simulink model "youhua_1226"  (R2017b)
settings: Solver=ode1  StartTime=0.0  StopTime=Inf  FixedStep=0.0002  RelTol=1e-3
PreLoadFcn:
  | initFun_4P.m
PostLoadFcn:
  | , if any(exist('dsrtsu_mdlpostloadfcn', 'file') == [2, 3, 6]), try dsrtsu_mdlpostloadfcn('Execute', bdroot); catch fprintf('Error in PostLoadFcn (dsrtsu_mdlpostloadfcn) for model "%s":\n %s\n', bdroot, lasterr); end, end,
InitFcn:
  | initFun_4P
undefined symbols (not defined in the file): CMAES_B_initial, CMAES_C_initial, CMAES_chiN_initial, CMAES_counteval_initial, CMAES_D_initial, CMAES_eigeneval_initial, CMAES_invsqrtC_initial, CMAES_pc_initial, CMAES_ps_initial, CMAES_sigma_initial, CMAES_xmean_initial
libraries: rti1202lib_adc_class1 x20, simulink x8, dsparch4 x6, rti1202serlib x4, rti1202lib_dio_class1 x4, dsextras x3, rtiemclib x2, rti1202lib_dac_class1 x1, rtitasklib x1
(part 3 of 6)

== system youhua_1226/DSpace Sensor Raw Readings/Digital Pins ==
  Constant : Constant  OutDataTypeStr=boolean
  DIO_CLASS1_BIT_IN_BL2 : rti1202lib_dio_class1/DIO_CLASS1_BIT_IN_BL1  DSProperties=struct('RTI',struct('Version',uint32(1),'BlockType',struct('isSLSource',uint8(1),'isSLSink',uint8(0),'isHWSource',uint8(1),'isHWSink',uint8(0),'isSetup',uint8(0),'isInline',uint8(1),'isNonInline',uint8(0),'isInterrupt',uint8(0),'isChannelwise',uint8(1)),'IOBoardType',{{'DS120X','STD','DIOC1'}},'UnitType','BIT','Identifier','BITIN','DialogType','ML','BlockSet','NONE','SlaveProcessor','NONE'))  RTIBlockInterface=struct('OutputPortsWidth',int32(1),'OutputPortsDataType',{{'SS_BOOLEAN'}},'OutputPortsActive',1,'OutputPortsName',{{'Out'}},'BlockDisplay',{{['DIO CL1 BIT IN\nPort: 1\nChannel: 1\nNumber of channels: 1'],'center'}},'IconTransparency','on','InitLevel',3,'DialogFcn','rti120xstddioc1bitingui','BlockName',struct('Token',{{'DIO_CLASS1_BIT_IN_BL1'}}))  RTIBlockParameters=struct('PortNo',{{1,'OFF',[]}},'ChannelNo',{{1,'OFF',[]}},'ChannelNumOf',{{1,'OFF',[]}},'EnableNoiseFilter',{{0,'OFF',[0 1]}},'FilterInterval',{{'0','OFF',[0 0.01]}},'FilterIntervalCheck',{{logical(0),'OFF',[]}},'EnableEvent',{{0,'OFF',[0 1]}},'EventMode',{{1,'OFF',[1 3]}},'EventOnFalling',{{1,'OFF',[0 1]}},'EventOnRising',{{0,'OFF',[0 1]}},'EventDelay',{{'0','OFF',[0 1.34]}},'EventRate',{{'1','OFF',[1 256]}},'EventBuildCheck',{{logical(0),'OFF',[]}},'TriggerLine',{{1,'OFF',[1 16]}},'EventChannelNoIdx',{{1,'OFF',[1 16]}},'TLCFileName',{{'rti120xdio_c1_bit_in','OFF',[]}})  RTISFcnParameters=struct('PortNo','int16','ChannelNo','int16','ChannelNumOf','int16','EnableNoiseFilter','int16','FilterInterval','double','EnableEvent','int16','EventMode','int16','EventOnFalling','int16','EventOnRising','int16','EventDelay','double','EventRate','int16','TriggerLine','int16','EventChannelNoIdx','int16','TLCFileName','char')  RTIBlockParaDefault=struct('PortNo',1,'ChannelNo',1,'ChannelNumOf',1,'EnableNoiseFilter',0,'FilterInterval',0,'FilterIntervalCheck',0,'EnableEvent',0,'EventMode',1,'EventOnFalling',1,'EventOnRising',0,'EventDelay',0,'EventRate',1,'EventBuildCheck',0,'TriggerLine',1,'EventChannelNoIdx',1,'TLCFileName','rti120xdio_c1_bit_in')
  DIO_CLASS1_BIT_OUT_BL1 : rti1202lib_dio_class1/DIO_CLASS1_BIT_OUT_BL1  DSProperties=struct('RTI',struct('Version',uint32(1),'BlockType',struct('isSLSource',uint8(0),'isSLSink',uint8(1),'isHWSource',uint8(0),'isHWSink',uint8(1),'isSetup',uint8(0),'isInline',uint8(1),'isNonInline',uint8(0),'isInterrupt',uint8(0),'isChannelwise',uint8(1)),'IOBoardType',{{'DS120X','STD','DIOC1'}},'UnitType','BIT','Identifier','BITOUT','DialogType','ML','BlockSet','NONE','SlaveProcessor','NONE'))  RTIBlockInterface=struct('InputPortsWidth',int32(1),'InputPortsActive',1,'InputPortsDataType',{{'SS_BOOLEAN'}},'InputPortsName',{{'In'}},'BlockDisplay',{{['DIO CL1 BIT OUT\nPort: 1\nChannel: 2\nNumber of channels: 1'],'center\'}},'IconTransparency','on','InitLevel',3,'DialogFcn','rti120xstddioc1bitoutgui','BlockName',struct('Token',{{'DIO_CLASS1_BIT_OUT_BL1'}}))  RTIBlockParameters=struct('PortNo',{{1,'OFF',[]}},'ChannelNo',{{2,'OFF',[]}},'ChannelNumOf',{{1,'OFF',[]}},'HighLevel',{{3,'OFF',[1 3]}},'OutputStateInit',{{zeros(1,16),'OFF',[0 1]}},'OutputStateTerm',{{zeros(1,16),'OFF',[0 1]}},'TerminationMode',{{0,'OFF',[0 1]}},'OutputStateTermValidate',{{0,'OFF',[0 1]}},'OutputStateInitSetAll',{{0,'OFF',[0 1]}},'OutputStateTermSetAll',{{0,'OFF',[0 1]}},'EnableEvent',{{0,'OFF',[0 1]}},'EventMode',{{1,'OFF',[1 3]}},'EventOnFalling',{{1,'OFF',[0 1]}},'EventOnRising',{{0,'OFF',[0 1]}},'EventDelay',{{'0','OFF',[0 1.34]}},'EventRate',{{'1','OFF',[1 256]}},'EventBuildCheck',{{logical(0),'OFF',[]}},'TriggerLine',{{1,'OFF',[1 16]}},'EventChannelNoIdx',{{1,'OFF',[1 16]}},'TLCFileName',{{'rti120xdio_c1_bit_out','OFF',[]}})  RTISFcnParameters=struct('PortNo','int16','ChannelNo','int16','ChannelNumOf','int16','HighLevel','int16','OutputStateInit','int16','OutputStateTerm','int16','TerminationMode','int16','OutputStateTermValidate','int16','EnableEvent','int16','EventMode','int16','EventOnFalling','int16','EventOnRising','int16','EventDelay','double','EventRate','int16','TriggerLine','int16','EventChannelNoIdx','int16','TLCFileName','char')  RTIBlockParaDefault=struct('PortNo',1,'ChannelNo',1,'ChannelNumOf',1,'HighLevel',1,'OutputStateInit',zeros(1,16),'OutputStateTerm',zeros(1,16),'TerminationMode',0,'OutputStateTermValidate',0,'OutputStateInitSetAll',0,'OutputStateTermSetAll',0,'EnableEvent',0,'EventMode',1,'EventOnFalling',1,'EventOnRising',0,'EventDelay',0,'EventRate',1,'EventBuildCheck',0,'TriggerLine',1,'EventChannelNoIdx',1,'TLCFileName','rti120xdio_c1_bit_out')
  Data Type Conversion : DataTypeConversion  OutDataTypeStr=double
  Out1 : Outport
  wires:
  DIO_CLASS1_BIT_IN_BL2/1 -> Data Type Conversion/1
  Constant/1 -> DIO_CLASS1_BIT_OUT_BL1/1
  Data Type Conversion/1 -> Out1/1

== system youhua_1226/DSpace Sensor Raw Readings/Encoder Readings ==
  EMC_ENCODER_BL2 : rtiemclib/EMC_ENCODER_BL1  DSProperties=struct('RTI',struct('Version',uint32(2),'BlockType',struct('isSLSource',uint8(1),'isSLSink',uint8(0),'isHWSource',uint8(1),'isHWSink',uint8(0),'isSetup',uint8(0),'isInline',uint8(1),'isNonInline',uint8(0),'isInterrupt',uint8(0),'isChannelwise',uint8(1)),'IOBoardType','DSEMC','UnitType','ENCODER','Identifier','ENCODER','DialogType','ML','BlockSet','RTIEMC','SlaveProcessor','NONE'))  RTIBlockInterface=struct('OutputPortsWidth',int32([1 1 1]),'OutputPortsActive',int32([1 1 0]),'OutputPortsName',{{'Position','Speed',['Index Detected']}},'OutputPortsDataType',{{'SS_DOUBLE','SS_DOUBLE','SS_BOOLEAN'}},'InitLevel',3,'IconTransparency','on','BlockDisplay',{{['EMC Encoder\nUnit: 1\nDIO class: 2\nPort: 1\nChannel: 1'],'center'}},'DialogFcn','rtiemcencodergui','BlockName',struct('Token',{{'EMC_ENCODER_BL1'}}))  RTIBlockParameters=struct('UnitNo',{{1,'OFF',[1 6]}},'DioClassNo',{{2,'OFF',[1 2]}},'PortNo',{{1,'OFF',[1 1]}},'ChannelNo',{{1,'OFF',[1 11]}},'HwSignalPin',{{['DIO1 ch1'],'OFF',[]}},'HwRefPin',{{'GND','OFF',[]}},'EnablePosMeasurement',{{1,'OFF',[0 1]}},'IndexSetMode',{{1,'OFF',[1 3]}},'EnableMinSpeed',{{1,'OFF',[0 1]}},'NumOfLines',{{'1250','OFF',[1 2097152]}},'InitAngleValue',{{'60','OFF',[0 359.99999]}},'IndexAngleValue',{{'0','OFF',[0 359.99999]}},'MinSpeedAngleValue',{{'45','OFF',[0.04 10000]}},'MinPosValue',{{'-125000','OFF',[-2097152 2097150.75]}},'MaxPosValue',{{'125000','OFF',[-2097151 2097151.75]}},'InitPosValue',{{'0','OFF',[-2097152 2097151.75]}},'IndexPosValue',{{'0','OFF',[-2097152 2097151.75]}},'MinSpeedPosValue',{{'1','OFF',[1 1000000]}},'IndexGateMode',{{1,'OFF',[0 1]}},'EnableNoiseFilter',{{0,'OFF',[0 1]}},'FilterInterval',{{'0','OFF',[0 0.01]}},'IndexDetectedOutPortMode',{{1,'OFF',[0 1]}},'BuildCheckAngleMeasurement',{{0,'OFF',[0 1]}},'BuildCheckAngleIndexMode',{{0,'OFF',[0 1]}},'BuildCheckPosIndexMode',{{0,'OFF',[0 1]}},'BuildCheckAngleMinSpeed',{{0,'OFF',[0 1]}},'BuildCheckPosMinSpeed',{{1,'OFF',[0 1]}},'TLCFileName',{{'rtiemcencoder','OFF',[]}})  RTISFcnParameters=struct('UnitNo','int32','DioClassNo','int32','PortNo','int32','ChannelNo','int32','EnablePosMeasurement','int32','IndexSetMode','int32','IndexDetectedOutPortMode','int32','EnableMinSpeed','int32','NumOfLines','uint32','InitAngleValue','double','IndexAngleValue','double','MinSpeedAngleValue','double','MinPosValue','double','MaxPosValue','double','InitPosValue','double','IndexPosValue','double','MinSpeedPosValue','double','IndexGateMode','int32','EnableNoiseFilter','int32','FilterInterval','double','TLCFileName','char')  RTIBlockParaDefault=struct('UnitNo',1,'DioClassNo',1,'PortNo',1,'ChannelNo',1,'HwSignalPin',['DIO1 ch1'],'HwRefPin','GND','EnablePosMeasurement',0,'IndexSetMode',1,'EnableMinSpeed',0,'NumOfLines',1024,'InitAngleValue',60,'IndexAngleValue',0,'MinSpeedAngleValue',45,'MinPosValue',0,'MaxPosValue',1023.75,'InitPosValue',0,'IndexPosValue',0,'MinSpeedPosValue',100,'IndexGateMode',0,'EnableNoiseFilter',0,'FilterInterval',0,'IndexDetectedOutPortMode',0,'BuildCheckAngleMeasurement',1,'BuildCheckAngleIndexMode',0,'BuildCheckPosIndexMode',0,'BuildCheckAngleMinSpeed',0,'BuildCheckPosMinSpeed',0,'TLCFileName','rtiemcencoder')
      settings: SourceProductName=dSPACE RTI Electric Motor Control Blockset
  EMC_ENCODER_BL4 : rtiemclib/EMC_ENCODER_BL1  DSProperties=struct('RTI',struct('Version',uint32(2),'BlockType',struct('isSLSource',uint8(1),'isSLSink',uint8(0),'isHWSource',uint8(1),'isHWSink',uint8(0),'isSetup',uint8(0),'isInline',uint8(1),'isNonInline',uint8(0),'isInterrupt',uint8(0),'isChannelwise',uint8(1)),'IOBoardType','DSEMC','UnitType','ENCODER','Identifier','ENCODER','DialogType','ML','BlockSet','RTIEMC','SlaveProcessor','NONE'))  RTIBlockInterface=struct('OutputPortsWidth',int32([1 1 1]),'OutputPortsActive',int32([1 1 0]),'OutputPortsName',{{'Position','Speed',['Index Detected']}},'OutputPortsDataType',{{'SS_DOUBLE','SS_DOUBLE','SS_BOOLEAN'}},'InitLevel',3,'IconTransparency','on','BlockDisplay',{{['EMC Encoder\nUnit: 3\nDIO class: 2\nPort: 1\nChannel: 5'],'center'}},'DialogFcn','rtiemcencodergui','BlockName',struct('Token',{{'EMC_ENCODER_BL1'}}))  RTIBlockParameters=struct('UnitNo',{{3,'OFF',[1 6]}},'DioClassNo',{{2,'OFF',[1 2]}},'PortNo',{{1,'OFF',[1 1]}},'ChannelNo',{{5,'OFF',[1 11]}},'HwSignalPin',{{['DIO1 ch1'],'OFF',[]}},'HwRefPin',{{'GND','OFF',[]}},'EnablePosMeasurement',{{1,'OFF',[0 1]}},'IndexSetMode',{{1,'OFF',[1 3]}},'EnableMinSpeed',{{1,'OFF',[0 1]}},'NumOfLines',{{'1250','OFF',[1 2097152]}},'InitAngleValue',{{'60','OFF',[0 359.99999]}},'IndexAngleValue',{{'0','OFF',[0 359.99999]}},'MinSpeedAngleValue',{{'45','OFF',[0.04 10000]}},'MinPosValue',{{'-125000','OFF',[-2097152 2097150.75]}},'MaxPosValue',{{'125000','OFF',[-2097151 2097151.75]}},'InitPosValue',{{'0','OFF',[-2097152 2097151.75]}},'IndexPosValue',{{'0','OFF',[-2097152 2097151.75]}},'MinSpeedPosValue',{{'1','OFF',[1 1000000]}},'IndexGateMode',{{1,'OFF',[0 1]}},'EnableNoiseFilter',{{0,'OFF',[0 1]}},'FilterInterval',{{'0','OFF',[0 0.01]}},'IndexDetectedOutPortMode',{{1,'OFF',[0 1]}},'BuildCheckAngleMeasurement',{{0,'OFF',[0 1]}},'BuildCheckAngleIndexMode',{{0,'OFF',[0 1]}},'BuildCheckPosIndexMode',{{0,'OFF',[0 1]}},'BuildCheckAngleMinSpeed',{{0,'OFF',[0 1]}},'BuildCheckPosMinSpeed',{{1,'OFF',[0 1]}},'TLCFileName',{{'rtiemcencoder','OFF',[]}})  RTISFcnParameters=struct('UnitNo','int32','DioClassNo','int32','PortNo','int32','ChannelNo','int32','EnablePosMeasurement','int32','IndexSetMode','int32','IndexDetectedOutPortMode','int32','EnableMinSpeed','int32','NumOfLines','uint32','InitAngleValue','double','IndexAngleValue','double','MinSpeedAngleValue','double','MinPosValue','double','MaxPosValue','double','InitPosValue','double','IndexPosValue','double','MinSpeedPosValue','double','IndexGateMode','int32','EnableNoiseFilter','int32','FilterInterval','double','TLCFileName','char')  RTIBlockParaDefault=struct('UnitNo',1,'DioClassNo',1,'PortNo',1,'ChannelNo',1,'HwSignalPin',['DIO1 ch1'],'HwRefPin','GND','EnablePosMeasurement',0,'IndexSetMode',1,'EnableMinSpeed',0,'NumOfLines',1024,'InitAngleValue',60,'IndexAngleValue',0,'MinSpeedAngleValue',45,'MinPosValue',0,'MaxPosValue',1023.75,'InitPosValue',0,'IndexPosValue',0,'MinSpeedPosValue',100,'IndexGateMode',0,'EnableNoiseFilter',0,'FilterInterval',0,'IndexDetectedOutPortMode',0,'BuildCheckAngleMeasurement',1,'BuildCheckAngleIndexMode',0,'BuildCheckPosIndexMode',0,'BuildCheckAngleMinSpeed',0,'BuildCheckPosMinSpeed',0,'TLCFileName','rtiemcencoder')
      settings: SourceProductName=dSPACE RTI Electric Motor Control Blockset
  Encoder Power Setup1 : rti1202lib_dio_class1/DIO_CLASS1_BIT_OUT_BL1  DSProperties=struct('RTI',struct('Version',uint32(1),'BlockType',struct('isSLSource',uint8(0),'isSLSink',uint8(1),'isHWSource',uint8(0),'isHWSink',uint8(1),'isSetup',uint8(0),'isInline',uint8(1),'isNonInline',uint8(0),'isInterrupt',uint8(0),'isChannelwise',uint8(1)),'IOBoardType',{{'DS120X','STD','DIOC1'}},'UnitType','BIT','Identifier','BITOUT','DialogType','ML','BlockSet','NONE','SlaveProcessor','NONE'))  RTIBlockInterface=struct('InputPortsWidth',int32(1),'InputPortsActive',1,'InputPortsDataType',{{'SS_BOOLEAN'}},'InputPortsName',{{'In'}},'BlockDisplay',{{['DIO CL1 BIT OUT\nPort: 3\nChannel: 11\nNumber of channels: 1'],'center\'}},'IconTransparency','on','InitLevel',3,'DialogFcn','rti120xstddioc1bitoutgui','BlockName',struct('Token',{{'DIO_CLASS1_BIT_OUT_BL1'}}))  RTIBlockParameters=struct('PortNo',{{3,'OFF',[]}},'ChannelNo',{{11,'OFF',[]}},'ChannelNumOf',{{1,'OFF',[]}},'HighLevel',{{3,'OFF',[1 3]}},'OutputStateInit',{{zeros(1,16),'OFF',[0 1]}},'OutputStateTerm',{{zeros(1,16),'OFF',[0 1]}},'TerminationMode',{{0,'OFF',[0 1]}},'OutputStateTermValidate',{{0,'OFF',[0 1]}},'OutputStateInitSetAll',{{0,'OFF',[0 1]}},'OutputStateTermSetAll',{{0,'OFF',[0 1]}},'EnableEvent',{{0,'OFF',[0 1]}},'EventMode',{{1,'OFF',[1 3]}},'EventOnFalling',{{1,'OFF',[0 1]}},'EventOnRising',{{0,'OFF',[0 1]}},'EventDelay',{{'0','OFF',[0 1.34]}},'EventRate',{{'1','OFF',[1 256]}},'EventBuildCheck',{{logical(0),'OFF',[]}},'TriggerLine',{{1,'OFF',[1 16]}},'EventChannelNoIdx',{{1,'OFF',[1 16]}},'TLCFileName',{{'rti120xdio_c1_bit_out','OFF',[]}})  RTISFcnParameters=struct('PortNo','int16','ChannelNo','int16','ChannelNumOf','int16','HighLevel','int16','OutputStateInit','int16','OutputStateTerm','int16','TerminationMode','int16','OutputStateTermValidate','int16','EnableEvent','int16','EventMode','int16','EventOnFalling','int16','EventOnRising','int16','EventDelay','double','EventRate','int16','TriggerLine','int16','EventChannelNoIdx','int16','TLCFileName','char')  RTIBlockParaDefault=struct('PortNo',1,'ChannelNo',1,'ChannelNumOf',1,'HighLevel',1,'OutputStateInit',zeros(1,16),'OutputStateTerm',zeros(1,16),'TerminationMode',0,'OutputStateTermValidate',0,'OutputStateInitSetAll',0,'OutputStateTermSetAll',0,'EnableEvent',0,'EventMode',1,'EventOnFalling',1,'EventOnRising',0,'EventDelay',0,'EventRate',1,'EventBuildCheck',0,'TriggerLine',1,'EventChannelNoIdx',1,'TLCFileName','rti120xdio_c1_bit_out')
  Encoder Power Setup3 : rti1202lib_dio_class1/DIO_CLASS1_BIT_OUT_BL1  DSProperties=struct('RTI',struct('Version',uint32(1),'BlockType',struct('isSLSource',uint8(0),'isSLSink',uint8(1),'isHWSource',uint8(0),'isHWSink',uint8(1),'isSetup',uint8(0),'isInline',uint8(1),'isNonInline',uint8(0),'isInterrupt',uint8(0),'isChannelwise',uint8(1)),'IOBoardType',{{'DS120X','STD','DIOC1'}},'UnitType','BIT','Identifier','BITOUT','DialogType','ML','BlockSet','NONE','SlaveProcessor','NONE'))  RTIBlockInterface=struct('InputPortsWidth',int32(1),'InputPortsActive',1,'InputPortsDataType',{{'SS_BOOLEAN'}},'InputPortsName',{{'In'}},'BlockDisplay',{{['DIO CL1 BIT OUT\nPort: 3\nChannel: 13\nNumber of channels: 1'],'center\'}},'IconTransparency','on','InitLevel',3,'DialogFcn','rti120xstddioc1bitoutgui','BlockName',struct('Token',{{'DIO_CLASS1_BIT_OUT_BL1'}}))  RTIBlockParameters=struct('PortNo',{{3,'OFF',[]}},'ChannelNo',{{13,'OFF',[]}},'ChannelNumOf',{{1,'OFF',[]}},'HighLevel',{{3,'OFF',[1 3]}},'OutputStateInit',{{zeros(1,16),'OFF',[0 1]}},'OutputStateTerm',{{zeros(1,16),'OFF',[0 1]}},'TerminationMode',{{0,'OFF',[0 1]}},'OutputStateTermValidate',{{0,'OFF',[0 1]}},'OutputStateInitSetAll',{{0,'OFF',[0 1]}},'OutputStateTermSetAll',{{0,'OFF',[0 1]}},'EnableEvent',{{0,'OFF',[0 1]}},'EventMode',{{1,'OFF',[1 3]}},'EventOnFalling',{{1,'OFF',[0 1]}},'EventOnRising',{{0,'OFF',[0 1]}},'EventDelay',{{'0','OFF',[0 1.34]}},'EventRate',{{'1','OFF',[1 256]}},'EventBuildCheck',{{logical(0),'OFF',[]}},'TriggerLine',{{1,'OFF',[1 16]}},'EventChannelNoIdx',{{1,'OFF',[1 16]}},'TLCFileName',{{'rti120xdio_c1_bit_out','OFF',[]}})  RTISFcnParameters=struct('PortNo','int16','ChannelNo','int16','ChannelNumOf','int16','HighLevel','int16','OutputStateInit','int16','OutputStateTerm','int16','TerminationMode','int16','OutputStateTermValidate','int16','EnableEvent','int16','EventMode','int16','EventOnFalling','int16','EventOnRising','int16','EventDelay','double','EventRate','int16','TriggerLine','int16','EventChannelNoIdx','int16','TLCFileName','char')  RTIBlockParaDefault=struct('PortNo',1,'ChannelNo',1,'ChannelNumOf',1,'HighLevel',1,'OutputStateInit',zeros(1,16),'OutputStateTerm',zeros(1,16),'TerminationMode',0,'OutputStateTermValidate',0,'OutputStateInitSetAll',0,'OutputStateTermSetAll',0,'EnableEvent',0,'EventMode',1,'EventOnFalling',1,'EventOnRising',0,'EventDelay',0,'EventRate',1,'EventBuildCheck',0,'TriggerLine',1,'EventChannelNoIdx',1,'TLCFileName','rti120xdio_c1_bit_out')
  VCC1 : Constant  OutDataTypeStr=boolean
  VCC3 : Constant  OutDataTypeStr=boolean
  Encoder_Position_1 : Outport
  Encoder_Speed_1 : Outport  Port=2
  Encoder_Position_3 : Outport  Port=3
  Encoder_Speed_3 : Outport  Port=4
  wires:
  EMC_ENCODER_BL2/2 -> Encoder_Speed_1/1
  EMC_ENCODER_BL2/1 -> Encoder_Position_1/1
  VCC1/1 -> Encoder Power Setup1/1
  VCC3/1 -> Encoder Power Setup3/1
  EMC_ENCODER_BL4/1 -> Encoder_Position_3/1
  EMC_ENCODER_BL4/2 -> Encoder_Speed_3/1

== system youhua_1226/RTI Data/RTI Data Store ==
  RTI Data Store : Subsystem  mask(RTI_DATA_STORE){}
      mask help:
      | RTI Data Store Block. This block is used by RTI to store internal model dependent data. Deleting this block will result in data loss.
      |
      | NEVER DELETE, COPY, OR MODIFY THIS BLOCK!
      mask Help:
      | RTI Data Store Block. This block is used by RTI to store internal model dependent data. Deleting this block will result in data loss.
      | 
      | NEVER DELETE, COPY, OR MODIFY THIS BLOCK!
      mask Display: text(0.5, 0.5, ' ', 'HorizontalAlignment', 'center');

== system youhua_1226/Sensor Data Conversion/get ankle vel ==
  position : Inport
  0.4low1 : DiscreteFilter  Numerator=|  Denominator=|
      Numerator=|
      | [   0.001567010350588   0.004701031051765   0.004701031051765   0.001567010350588
      | ]
      Denominator=|
      | [   1.000000000000000  -2.498608344691178   2.115254127003159  -0.604109699507275
      | ]
  Discrete Derivative : simulink/Discrete/Discrete Derivative  gainval=1.0  ICPrevScaledInput=0.0  InputProcessing=Inherited  OutMin=[]  OutMax=[]  OutDataType=fixdt(1, 16)  OutScaling=2^-10  DoSatur=off
  velocity : Outport
  raw velocity : Outport  Port=2
  wires:
  Discrete Derivative/1 -> raw velocity/1, 0.4low1/1
  position/1 -> Discrete Derivative/1
  0.4low1/1 -> velocity/1

== system youhua_1226/Sensor Data Conversion/get force vel ==
  position : Inport
  0.4low1 : DiscreteFilter  Numerator=|  Denominator=|
      Numerator=|
      | [   0.001567010350588   0.004701031051765   0.004701031051765   0.001567010350588
      | ]
      Denominator=|
      | [   1.000000000000000  -2.498608344691178   2.115254127003159  -0.604109699507275
      | ]
  Discrete Derivative : simulink/Discrete/Discrete Derivative  gainval=1.0  ICPrevScaledInput=0.0  InputProcessing=Inherited  OutMin=[]  OutMax=[]  OutDataType=fixdt(1, 16)  OutScaling=2^-10  DoSatur=off
  velocity : Outport
  raw velocity : Outport  Port=2
  wires:
  Discrete Derivative/1 -> raw velocity/1, 0.4low1/1
  position/1 -> Discrete Derivative/1
  0.4low1/1 -> velocity/1

== system youhua_1226/Sensor Data Conversion/get motor acc ==
  position : Inport
  0.4low1 : DiscreteFilter  Numerator=|  Denominator=|
      Numerator=|
      | [   0.001567010350588   0.004701031051765   0.004701031051765   0.001567010350588
      | ]
      Denominator=|
      | [   1.000000000000000  -2.498608344691178   2.115254127003159  -0.604109699507275
      | ]
  Discrete Derivative : simulink/Discrete/Discrete Derivative  gainval=1.0  ICPrevScaledInput=0.0  InputProcessing=Inherited  OutMin=[]  OutMax=[]  OutDataType=fixdt(1, 16)  OutScaling=2^-10  DoSatur=off
  velocity : Outport
  raw velocity : Outport  Port=2
  wires:
  position/1 -> Discrete Derivative/1
  Discrete Derivative/1 -> raw velocity/1, 0.4low1/1
  0.4low1/1 -> velocity/1

== system youhua_1226/Sensor Data Conversion/get motor vel ==
  position : Inport
  0.4low1 : DiscreteFilter  Numerator=|  Denominator=|
      Numerator=|
      | [   0.001567010350588   0.004701031051765   0.004701031051765   0.001567010350588
      | ]
      Denominator=|
      | [   1.000000000000000  -2.498608344691178   2.115254127003159  -0.604109699507275
      | ]
  Discrete Derivative : simulink/Discrete/Discrete Derivative  gainval=1.0  ICPrevScaledInput=0.0  InputProcessing=Inherited  OutMin=[]  OutMax=[]  OutDataType=fixdt(1, 16)  OutScaling=2^-10  DoSatur=off
  velocity : Outport
  raw velocity : Outport  Port=2
  wires:
  position/1 -> Discrete Derivative/1
  Discrete Derivative/1 -> raw velocity/1, 0.4low1/1
  0.4low1/1 -> velocity/1

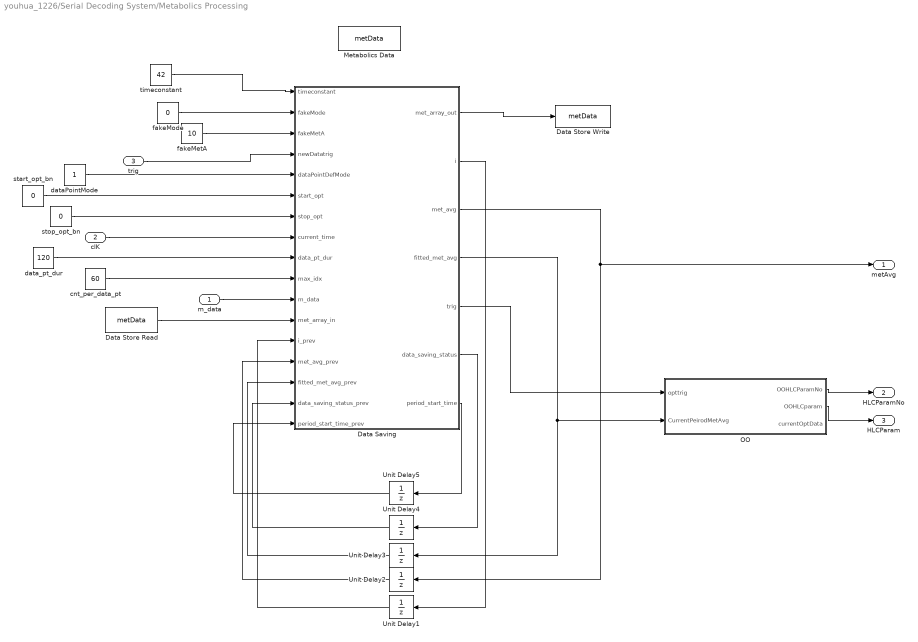
== system youhua_1226/Serial Decoding System/Metabolics Processing ==
  m_data : Inport
  clK : Inport  Port=2
  "trig " : Inport  Port=3
  Data Saving : MATLAB Function  TreatAsAtomicUnit=on
  Data Store Read : DataStoreRead  DataStoreName=metData
  Data Store Write : DataStoreWrite  DataStoreName=metData
  Metabolics Data : DataStoreMemory  DataStoreName=metData  ReadBeforeWriteMsg=warning  WriteAfterWriteMsg=warning  WriteAfterReadMsg=warning  InitialValue=zeros(2,200)  ShowAdditionalParam=off
  OO : Subsystem
  Unit Delay{1..5} (5 alike) : UnitDelay  SampleTime=-1
  cnt_per_data_pt : Constant  Value=60
  dataPointMode : Constant
  data_pt_dur : Constant  Value=120
  fakeMetA : Constant  Value=10
  fakeMode : Constant  Value=0
  start_opt_bn : Constant  Value=0
  stop_opt_bn : Constant  Value=0
  timeconstant : Constant  Value=42
  metAvg : Outport
  HLCParamNo : Outport  Port=2
  HLCParam : Outport  Port=3
  wires:
  m_data/1 -> Data Saving/11(m_data)
  Unit Delay1/1 -> Data Saving/13(i_prev)
  Data Store Read/1 -> Data Saving/12(met_array_in)
  Data Saving/1(met_array_out) -> Data Store Write/1
  cnt_per_data_pt/1 -> Data Saving/10(max_idx)
  Data Saving/2(i) -> Unit Delay1/1
  Data Saving/3(met_avg) -> Unit Delay2/1, metAvg/1
  Unit Delay2/1 -> Data Saving/14(met_avg_prev)
  OO/2(OOHLCparam) -> HLCParam/1
  Data Saving/5(trig) -> OO/1(opttrig)
  OO/1(OOHLCParamNo) -> HLCParamNo/1
  clK/1 -> Data Saving/8(current_time)
  data_pt_dur/1 -> Data Saving/9(data_pt_dur)
  start_opt_bn/1 -> Data Saving/6(start_opt)
  stop_opt_bn/1 -> Data Saving/7(stop_opt)
  Data Saving/6(data_saving_status) -> Unit Delay4/1
  Unit Delay4/1 -> Data Saving/16(data_saving_status_prev)
  dataPointMode/1 -> Data Saving/5(dataPointDefMode)
  Data Saving/7(period_start_time) -> Unit Delay5/1
  Unit Delay5/1 -> Data Saving/17(period_start_time_prev)
  Unit Delay3/1 -> Data Saving/15(fitted_met_avg_prev)
  Data Saving/4(fitted_met_avg) -> Unit Delay3/1, OO/2(CurrentPeirodMetAvg)
  "trig "/1 -> Data Saving/4(newDatatrig)
  fakeMode/1 -> Data Saving/2(fakeMode)
  fakeMetA/1 -> Data Saving/3(fakeMetA)
  timeconstant/1 -> Data Saving/1(timeconstant)

== system youhua_1226/Serial Decoding System/Serial ==
  Constant : Constant  OutDataTypeStr=uint32
  DS1202SER_RX_C1 : rti1202serlib/DS1202SER_RX_C1  Reserved1=[]  Reserved2=[]  Reserved3=[]  Reserved4=[]  DSProperties=struct('RTI',struct('IOBoardType',{{'DS1202','SER'}},'SlaveProcessor','NONE','Version',uint32(1),'BlockType',struct('isSLSource',uint8(1),'isSLSink',uint8(1),'isHWSource',uint8(0),'isHWSink',uint8(1),'isSetup',uint8(0),'isInline',uint8(1),'isNonInline',uint8(0),'isInterrupt',uint8(0),'isChannelwise',uint8(1)),'UnitType','GENSER','Identifier','RECEIVE','DialogType','ML','BlockSet','NONE'))  RTIBlockInterface=struct('BlockName',struct('Token',{{'DS1202SER_RX_C'}},'BlockParam',{{'ChannelNo'}}),'InputPortsWidth',int32(1),'InputPortsActive',1,'InputPortsDataType',{{'SS_UINT32'}},'InputPortsName',{{'NumBytes'}},'OutputPortsWidth',int32([1 1 1]),'OutputPortsActive',[1 1 1],'OutputPortsDataType',{{'SS_UINT8','SS_UINT32','SS_INT32'}},'OutputPortsName',{{'RXBytes','NumRXBytes','Status'}},'BlockDisplay',{{['Serial Receive'],'center'}},'IconTransparency','on','ParameterTunableNames',{{'BytesRefNumOf'}},'InitLevel',2,'DialogFcn','guigenserreceive','MaskDescription',['To read data from the UART SW FIFO.'])  RTIBlockParameters=struct('BoardNo',{{1,'ON',[1 1]}},'ChannelNo',{{1,'ON',[1 2]}},'ChannelNumOf',{{2,'OFF',[]}},'ReceptionDataMode',{{1,'OFF',[]}},'ParamTunableMode',{{1,'OFF',[]}},'BytesRefNumOfT',{{1,'OFF',[1 inf]}},'BytesRefNumOfNT',{{1,'OFF',[1 inf]}},'BytesRefNumOfMax',{{1,'OFF',[1 inf]}},'BytesRefNumOfMode',{{0,'OFF',[]}},'BytesActNumOfMode',{{1,'OFF',[]}},'ReceptionStatusMode',{{1,'OFF',[]}},'FifoSizeDefault',{{64,'OFF',[]}},'TLCFileName',{{'rtigenserreceive','OFF',[]}})  RTISFcnParameters=struct('BoardNo','double','ChannelNo','double','ChannelNumOf','double','ReceptionDataMode','double','ParamTunableMode','double','BytesRefNumOfT','double','BytesRefNumOfNT','double','BytesRefNumOfMax','double','BytesRefNumOfMode','double','BytesActNumOfMode','double','ReceptionStatusMode','double','TLCFileName','char')  RTIBlockParaDefault=struct('BoardNo',1,'ChannelNo',1,'ChannelNumOf',2,'ReceptionDataMode',1,'ParamTunableMode',1,'BytesRefNumOfT',1,'BytesRefNumOfNT',1,'BytesRefNumOfMax',1,'BytesRefNumOfMode',0,'BytesActNumOfMode',1,'ReceptionStatusMode',1,'FifoSizeDefault',64,'TLCFileName','rtigenserreceive')
  DS1202SER_SETUP_C1 : rti1202serlib/DS1202SER_SETUP_C1  Reserved1=[]  Reserved2=[]  Reserved3=[]  Reserved4=[]  DSProperties=struct('RTI',struct('Version',uint32(2),'IOBoardType',{{'DS1202','SER'}},'SlaveProcessor','NONE','BlockType',struct('isSLSource',uint8(0),'isSLSink',uint8(0),'isHWSource',uint8(0),'isHWSink',uint8(0),'isSetup',uint8(1),'isInline',uint8(1),'isNonInline',uint8(0),'isInterrupt',uint8(0),'isChannelwise',uint8(1)),'UnitType','GENSER','Identifier','SETUP','DialogType','ML','BlockSet','NONE'))  RTIBlockInterface=struct('BlockName',struct('Token',{{'DS1202SER_SETUP_C'}},'BlockParam',{{'ChannelNo'}}),'BlockDisplay',{{['Serial Setup'],'center'}},'IconTransparency','off','ParameterTunableNames',{{}},'InitLevel',1,'DialogFcn','guigensersetup','MaskDescription',['To set the global specifications for the UART interface.'])  RTIBlockParameters=struct('ParityMode',{{1,'OFF',[1 5]}},'TransceiverMode',{{[1;1],'OFF',[]}},'QuartzFrequency',{{160000000,'OFF',[]}},'BoardNo',{{1,'ON',[1 1]}},'ChannelNo',{{1,'ON',[1 2]}},'ChannelNumOf',{{2,'OFF',[]}},'BaudRate',{{115200,'OFF',[]}},'DataBitsNumOf',{{4,'OFF',[1 4]}},'StopBitsNumOf',{{1,'OFF',[1 3]}},'ReceiveIntLevelUart',{{4,'OFF',[1 4]}},'AutoflowMode',{{0,'OFF',[]}},'FifoSize',{{64,'OFF',[]}},'ReceiveIntLevelFifo',{{0,'OFF',[]}},'FifoOverrunMode',{{1,'OFF',[]}},'FifoBlockSize',{{0,'OFF',[]}},'TermMode',{{1,'OFF',[]}},'TLCFileName',{{'rtigensersetup','OFF',[]}})  RTISFcnParameters=struct('BoardNo','double','ChannelNo','double','ChannelNumOf','double','BaudRate','double','DataBitsNumOf','double','StopBitsNumOf','double','ParityMode','double','TransceiverMode','double','ReceiveIntLevelUart','double','AutoflowMode','double','FifoSize','double','ReceiveIntLevelFifo','double','FifoBlockSize','double','TermMode','double','QuartzFrequency','double','TLCFileName','char')  RTIBlockParaDefault=struct('ParityMode',1,'TransceiverMode',[1;1],'QuartzFrequency',160000000,'BoardNo',1,'ChannelNo',1,'ChannelNumOf',2,'BaudRate',115200,'DataBitsNumOf',4,'StopBitsNumOf',1,'ReceiveIntLevelUart',4,'AutoflowMode',0,'FifoSize',64,'ReceiveIntLevelFifo',0,'FifoOverrunMode',1,'FifoBlockSize',0,'TermMode',1,'TLCFileName','rtigensersetup')
  DS1202SER_STAT_C1 : rti1202serlib/DS1202SER_STAT_C1  Reserved1=[]  Reserved2=[]  Reserved3=[]  Reserved4=[]  DSProperties=struct('RTI',struct('IOBoardType',{{'DS1202','SER'}},'SlaveProcessor','NONE','Version',uint32(1),'BlockType',struct('isSLSource',uint8(1),'isSLSink',uint8(0),'isHWSource',uint8(0),'isHWSink',uint8(0),'isSetup',uint8(0),'isInline',uint8(1),'isNonInline',uint8(0),'isInterrupt',uint8(0),'isChannelwise',uint8(1)),'UnitType','GENSER','Identifier','STATUS','DialogType','ML','BlockSet','NONE'))  RTIBlockInterface=struct('BlockName',struct('Token',{{'DS1202SER_STAT_C'}},'BlockParam',{{'ChannelNo'}}),'OutputPortsWidth',int32([8 8 8]),'OutputPortsActive',[1 1 1],'OutputPortsName',{{'Line','Modem','Interrupt'}},'OutputPortsDataType',{{'SS_BOOLEAN','SS_BOOLEAN','SS_BOOLEAN'}},'BlockDisplay',{{['Serial Status'],'left'}},'IconTransparency','on','ParameterTunableNames',{{}},'InitLevel',1,'DialogFcn','guigenserstatus','MaskDescription',['To read the contents of the UART status register.'])  RTIBlockParameters=struct('BoardNo',{{1,'ON',[1 1]}},'ChannelNo',{{1,'ON',[1 2]}},'ChannelNumOf',{{2,'OFF',[]}},'LineStatUartMode',{{1,'OFF',[]}},'ModemStatUartMode',{{1,'OFF',[]}},'InterruptStatUartMode',{{1,'OFF',[]}},'TLCFileName',{{'rtigenserstatus','OFF',[]}})  RTISFcnParameters=struct('BoardNo','double','ChannelNo','double','ChannelNumOf','double','LineStatUartMode','double','ModemStatUartMode','double','InterruptStatUartMode','double','TLCFileName','char')  RTIBlockParaDefault=struct('BoardNo',1,'ChannelNo',1,'ChannelNumOf',2,'LineStatUartMode',1,'ModemStatUartMode',1,'InterruptStatUartMode',1,'TLCFileName','rtigenserstatus')
  SerialReceived : Outport
  1 : Outport  Port=2
  2 : Outport  Port=3
  3 : Outport  Port=4
  4 : Outport  Port=5
  5 : Outport  Port=6
  wires:
  DS1202SER_RX_C1/1 -> SerialReceived/1
  Constant/1 -> DS1202SER_RX_C1/1
  DS1202SER_RX_C1/2 -> 1/1
  DS1202SER_RX_C1/3 -> 2/1
  DS1202SER_STAT_C1/1 -> 3/1
  DS1202SER_STAT_C1/2 -> 4/1
  DS1202SER_STAT_C1/3 -> 5/1

== system youhua_1226/CONTROL/Control and Display/LearningDataReset ==
  Trigger : TriggerPort  VariantControl=(inherit)
  filtered data store write : DataStoreWrite  DataStoreName=filteredStepData
  myinitialdata : Constant  Value=zeros(2,450)
  wires:
  myinitialdata/1 -> filtered data store write/1

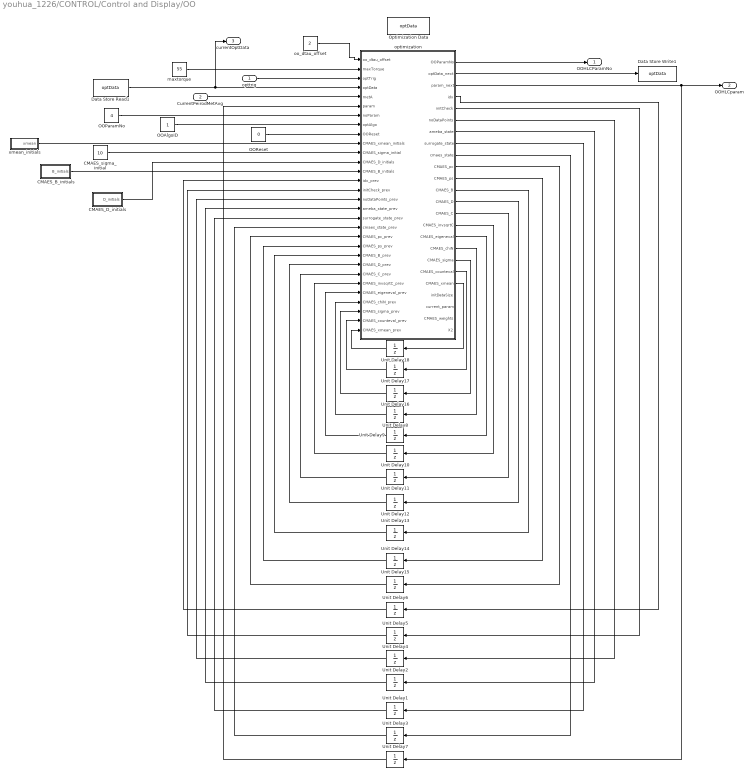
== system youhua_1226/CONTROL/Control and Display/OO ==
  opttrig : Inport
  CurrentPeirodMetAvg : Inport  Port=2
  CMAES_B_initials : Subsystem
  CMAES_D_initials : Subsystem
  CMAES_sigma_initial : Constant  Value=10
  Data Store Read1 : DataStoreRead  DataStoreName=optData
  Data Store Write1 : DataStoreWrite  DataStoreName=optData
  OOAlgoID : Constant
  OOParamNo : Constant  Value=4
  OOReset : Constant  Value=0
  Optimization Data : DataStoreMemory  DataStoreName=optData  ReadBeforeWriteMsg=warning  WriteAfterWriteMsg=warning  WriteAfterReadMsg=warning  InitialValue=zeros(8,5)  ShowAdditionalParam=off
  Unit Delay{1..6} (6 alike) : UnitDelay  SampleTime=-1
  Unit Delay10 : UnitDelay  InitialCondition=CMAES_invsqrtC_initial  SampleTime=-1
  Unit Delay11 : UnitDelay  InitialCondition=CMAES_C_initial  SampleTime=-1
  Unit Delay12 : UnitDelay  InitialCondition=CMAES_D_initial  SampleTime=-1
  Unit Delay13 : UnitDelay  InitialCondition=CMAES_B_initial  SampleTime=-1
  Unit Delay14 : UnitDelay  InitialCondition=CMAES_ps_initial  SampleTime=-1
  Unit Delay15 : UnitDelay  InitialCondition=CMAES_pc_initial  SampleTime=-1
  Unit Delay16 : UnitDelay  InitialCondition=CMAES_sigma_initial  SampleTime=-1
  Unit Delay17 : UnitDelay  InitialCondition=CMAES_counteval_initial  SampleTime=-1
  Unit Delay18 : UnitDelay  InitialCondition=CMAES_xmean_initial  SampleTime=-1
  Unit Delay7 : UnitDelay  InitialCondition=zeros(4,1)  SampleTime=-1
  Unit Delay8 : UnitDelay  InitialCondition=CMAES_chiN_initial  SampleTime=-1
  Unit Delay9 : UnitDelay  InitialCondition=CMAES_eigeneval_initial  SampleTime=-1
  maxtorque : Constant  Value=55
  oo_dtau_offset : Constant  Value=2
  optimization : MATLAB Function  TreatAsAtomicUnit=on
  xmean_initials : Subsystem
  OOHLCParamNo : Outport
  OOHLCparam : Outport  Port=2
  currentOptData : Outport  Port=3
  wires:
  Data Store Read1/1 -> optimization/4(optData), currentOptData/1
  OOAlgoID/1 -> optimization/8(optAlgo)
  CurrentPeirodMetAvg/1 -> optimization/5(metA)
  optimization/3(param_next) -> Unit Delay7/1, OOHLCparam/1
  optimization/2(optData_next) -> Data Store Write1/1
  optimization/1(OOParamNo) -> OOHLCParamNo/1
  OOParamNo/1 -> optimization/7(noParam)
  optimization/4(idx) -> Unit Delay6/1
  Unit Delay7/1 -> optimization/6(param)
  Unit Delay6/1 -> optimization/14(idx_prev)
  OOReset/1 -> optimization/9(OOReset)
  optimization/5(initCheck) -> Unit Delay5/1
  Unit Delay5/1 -> optimization/15(initCheck_prev)
  optimization/6(noDataPoints) -> Unit Delay4/1
  Unit Delay4/1 -> optimization/16(noDataPoints_prev)
  Unit Delay2/1 -> optimization/17(ameba_state_prev)
  optimization/7(ameba_state) -> Unit Delay2/1
  optimization/8(surrogate_state) -> Unit Delay1/1
  Unit Delay1/1 -> optimization/18(surrogate_state_prev)
  optimization/9(cmaes_state) -> Unit Delay3/1
  Unit Delay3/1 -> optimization/19(cmaes_state_prev)
  optimization/17(CMAES_chiN) -> Unit Delay8/1
  Unit Delay8/1 -> optimization/27(CMAES_chiN_prev)
  optimization/16(CMAES_eigeneval) -> Unit Delay9/1
  Unit Delay9/1 -> optimization/26(CMAES_eigeneval_prev)
  optimization/15(CMAES_invsqrtC) -> Unit Delay10/1
  Unit Delay10/1 -> optimization/25(CMAES_invsqrtC_prev)
  optimization/14(CMAES_C) -> Unit Delay11/1
  Unit Delay11/1 -> optimization/24(CMAES_C_prev)
  optimization/13(CMAES_D) -> Unit Delay12/1
  optimization/12(CMAES_B) -> Unit Delay13/1
  optimization/11(CMAES_ps) -> Unit Delay14/1
  optimization/10(CMAES_pc) -> Unit Delay15/1
  Unit Delay12/1 -> optimization/23(CMAES_D_prev)
  Unit Delay13/1 -> optimization/22(CMAES_B_prev)
  Unit Delay14/1 -> optimization/21(CMAES_ps_prev)
  Unit Delay15/1 -> optimization/20(CMAES_pc_prev)
  optimization/18(CMAES_sigma) -> Unit Delay16/1
  Unit Delay16/1 -> optimization/28(CMAES_sigma_prev)
  optimization/19(CMAES_counteval) -> Unit Delay17/1
  Unit Delay17/1 -> optimization/29(CMAES_counteval_prev)
  optimization/20(CMAES_xmean) -> Unit Delay18/1
  Unit Delay18/1 -> optimization/30(CMAES_xmean_prev)
  opttrig/1 -> optimization/3(optTrig)
  CMAES_sigma_initial/1 -> optimization/11(CMAES_sigma_initial)
  xmean_initials/1(xmean) -> optimization/10(CMAES_xmean_initials)
  CMAES_D_initials/1(D_initials) -> optimization/12(CMAES_D_initials)
  maxtorque/1 -> optimization/2(maxTorque)
  CMAES_B_initials/1(B_initials) -> optimization/13(CMAES_B_initials)
  oo_dtau_offset/1 -> optimization/1(oo_dtau_offset)

== system youhua_1226/CONTROL/Control and Display/OutputBlock ==
  state_params : Inport
  comm_vel : Inport  Port=2
  state_vars : Inport  Port=3
  Display and Recording : MATLAB Function  TreatAsAtomicUnit=on
  Mux : Mux  Inputs=53
  Terminator : Terminator
  wires:
  comm_vel/1 -> Display and Recording/3(motor_velocity)
  state_params/1 -> Display and Recording/1(current_state)
  state_vars/1 -> Display and Recording/2(state_variables)
  Display and Recording/1(state) -> Mux/1
  Display and Recording/2(desired_velocity) -> Mux/2
  Display and Recording/3(zero_ankle_pos) -> Mux/3
  Display and Recording/4(zero_motor_pos) -> Mux/4
  Display and Recording/5(ankle_pos) -> Mux/5
  Display and Recording/6(motor_pos) -> Mux/6
  Display and Recording/7(desired_torque) -> Mux/7
  Display and Recording/8(measured_torque) -> Mux/8
  Display and Recording/9(load_force) -> Mux/9
  Display and Recording/10(load_angle) -> Mux/10
  Display and Recording/11(load_pivot_distance) -> Mux/11
  Display and Recording/12(delta_motor_pos) -> Mux/12
  Display and Recording/13(slack_motor_pos) -> Mux/13
  Display and Recording/14(torque_error) -> Mux/14
  Display and Recording/15(Kp) -> Mux/15
  Display and Recording/16(ankle_vel) -> Mux/16
  Display and Recording/17(motor_vel) -> Mux/17
  Display and Recording/18(motor_acc) -> Mux/18
  Display and Recording/19(Kd) -> Mux/19
  Display and Recording/20(Ki) -> Mux/20
  Display and Recording/21(controller_type) -> Mux/21
  Display and Recording/22(Kc) -> Mux/22
  Display and Recording/23(current_time) -> Mux/23
  Display and Recording/24(state_start_time) -> Mux/24
  Display and Recording/25(curve_id) -> Mux/25
  Display and Recording/26(Kpp) -> Mux/26
  Display and Recording/27(accumulated_torque_error) -> Mux/27
  Display and Recording/28(desired_motor_pos) -> Mux/28
  Display and Recording/29(walk_control_mode) -> Mux/29
  Display and Recording/30(prev_step_accumulated_error) -> Mux/30
  Display and Recording/31(curr_step_accumulated_error) -> Mux/31
  Display and Recording/32(learning_control_input) -> Mux/32
  Display and Recording/33(learning_control_input2) -> Mux/33
  Display and Recording/34(Kp2) -> Mux/34
  Display and Recording/35(Kl) -> Mux/35
  Display and Recording/36(Kl2) -> Mux/36
  Display and Recording/37(flag_d_p) -> Mux/37
  Display and Recording/38(gamma) -> Mux/38
  Display and Recording/39(Lce) -> Mux/39
  Display and Recording/40(Lmtu) -> Mux/40
  Display and Recording/41(FL) -> Mux/41
  Display and Recording/42(Fpe) -> Mux/42
  Display and Recording/43(ACT) -> Mux/43
  Display and Recording/44(STIM) -> Mux/44
  Display and Recording/45(Fmtu) -> Mux/45
  Display and Recording/46(Lcedot) -> Mux/46
  Display and Recording/47(learned_value) -> Mux/47
  Display and Recording/48(learned_avg) -> Mux/48
  Display and Recording/49(accumulated_pos_error) -> Mux/49
  Display and Recording/50(gamma1) -> Mux/50
  Display and Recording/51(gamma2) -> Mux/51
  Display and Recording/52(gamma3) -> Mux/52
  Display and Recording/53(gamma4) -> Mux/53
  Mux/1 -> Terminator/1

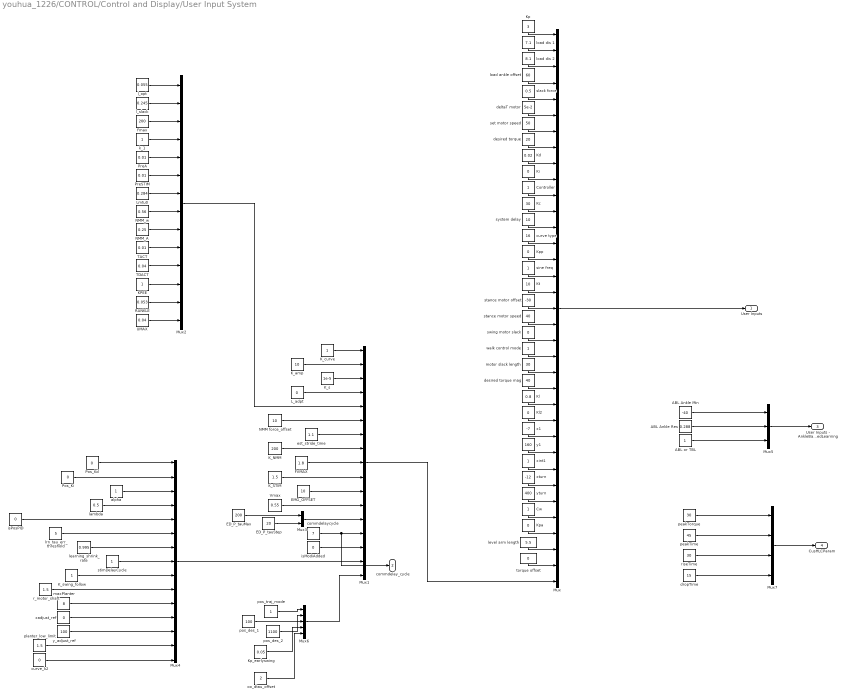
== system youhua_1226/CONTROL/Control and Display/User Input System ==
  ABL Ankle Min : Constant  Value=-40
  ABL Ankle Res : Constant  Value=0.288
  ABL or TBL : Constant
  Controller : Constant
  Cw : Constant
  ED_P_tauMax : Constant  Value=200
  ED_P_tauStep : Constant  Value=20
  EMG_OFFSET : Constant  Value=10
  FVMAX : Constant  Value=1.8
  Fmax : Constant  Value=200
  KPEE : Constant
  K_NMM : Constant  Value=200
  K_STIM : Constant  Value=1.5
  K_amp : Constant  Value=10
  K_curve : Constant
  K_s : Constant  Value=1e-5
  K_swing_follow : Constant
  Kc : Constant  Value=30
  Kd : Constant  Value=0.02
  Ki : Constant  Value=0
  Kl : Constant  Value=0.8
  Kl2 : Constant  Value=0
  Kp : Constant  Value=3
  Kp_earlyswing : Constant  Value=0.05
  Kpa : Constant  Value=0
  Kpp : Constant  Value=0
  Kt : Constant  Value=10
  L_adpt : Constant  Value=0
  Lmtu0 : Constant  Value=0.284
  Mux : Mux  Inputs=35
  Mux1 : Mux  Inputs=17
  Mux2 : Mux  Inputs=14
  Mux3 : Mux  Inputs=2
  Mux4 : Mux  Inputs=15
  Mux5 : Mux  Inputs=3
  Mux6 : Mux  Inputs=5
  Mux7 : Mux
  NMM force_offset : Constant  Value=10
  NMM_A : Constant  Value=0.25
  NMM_w : Constant  Value=0.56
  Pos_Kd : Constant  Value=0
  Pos_Ki : Constant  Value=0
  PreA : Constant  Value=0.01
  PreSTIM : Constant  Value=0.01
  RANKLE : Constant  Value=0.053
  TACT : Constant  Value=0.01
  TDACT : Constant  Value=0.04
  UMAX : Constant  Value=0.04
  Vmax : Constant  Value=0.55
  alpha : Constant
  commdelaycycle : Constant  Value=7
  curve type : Constant  Value=16
  curve_k2 : Constant  Value=0
  deltaT motor : Constant  Value=5e-2
  desired torque : Constant  Value=20
  desired torque mag : Constant  Value=40
  dropTime : Constant  Value=15
  est_stride_time : Constant  Value=1.1
  isModiAdded : Constant  Value=0
  isPosPID : Constant  Value=0
  k_1 : Constant
  l_opt : Constant  Value=0.055
  l_slack : Constant  Value=0.245
  lambda : Constant  Value=0.5
  learning_shrink_rate : Constant  Value=0.995
  level arm length : Constant  Value=5.5
  load ankle offset : Constant  Value=60
  load dis 1 : Constant  Value=7.1
  load dis 2 : Constant  Value=8.1
  lrn_tau_err_threshold : Constant  Value=5
  maxPlanter : Constant  Value=8
  motor slack length : Constant  Value=30
  oo_dtau_offset : Constant  Value=2
  peakTime : Constant  Value=45
  peakTorque : Constant  Value=30
  planter_low_limit : Constant  Value=1.5
  pos_des_1 : Constant  Value=100
  pos_des_2 : Constant  Value=1100
  pos_traj_mode : Constant
  r_motor_shaft : Constant  Value=1.5
  riseTime : Constant  Value=30
  set motor speed : Constant  Value=50
  sine freq : Constant
  slack force : Constant  Value=0.5
  stance motor offset : Constant  Value=-30
  stance motor speed : Constant  Value=40
  stimDelayCycle : Constant
  swing motor slack : Constant  Value=0
  system delay : Constant  Value=10
  torque offset : Constant  Value=0
  walk control mode : Constant
  x1 : Constant  Value=-7
  xadjust_ref : Constant  Value=0
  xint1 : Constant
  xturn : Constant  Value=-12
  y1 : Constant  Value=160
  y_adjust_ref : Constant  Value=100
  yturn : Constant  Value=400
  User Inputs : Outport
  commdelay_cycle : Outport  Port=2
  User Inputs - AnkleBasedLearning : Outport  Port=3
  CusHLCParam : Outport  Port=4
  wires:
  Kp/1 -> Mux/1
  load dis 1/1 -> Mux/2
  load dis 2/1 -> Mux/3
  load ankle offset/1 -> Mux/4
  slack force/1 -> Mux/5
  deltaT motor/1 -> Mux/6
  set motor speed/1 -> Mux/7
  desired torque/1 -> Mux/8
  Kd/1 -> Mux/9
  Ki/1 -> Mux/10
  Controller/1 -> Mux/11
  Kc/1 -> Mux/12
  system delay/1 -> Mux/13
  curve type/1 -> Mux/14
  Kpp/1 -> Mux/15
  sine freq/1 -> Mux/16
  Kt/1 -> Mux/17
  stance motor offset/1 -> Mux/18
  stance motor speed/1 -> Mux/19
  swing motor slack/1 -> Mux/20
  walk control mode/1 -> Mux/21
  motor slack length/1 -> Mux/22
  desired torque mag/1 -> Mux/23
  Kl/1 -> Mux/24
  Kl2/1 -> Mux/25
  x1/1 -> Mux/26
  y1/1 -> Mux/27
  xint1/1 -> Mux/28
  xturn/1 -> Mux/29
  yturn/1 -> Mux/30
  Cw/1 -> Mux/31
  Kpa/1 -> Mux/32
  level arm length/1 -> Mux/33
  torque offset/1 -> Mux/34
  Mux/1 -> User Inputs/1
  Mux1/1 -> Mux/35
  K_curve/1 -> Mux1/1
  K_amp/1 -> Mux1/2
  K_s/1 -> Mux1/3
  L_adpt/1 -> Mux1/4
  Mux2/1 -> Mux1/5
  l_opt/1 -> Mux2/1
  l_slack/1 -> Mux2/2
  Fmax/1 -> Mux2/3
  k_1/1 -> Mux2/4
  PreA/1 -> Mux2/5
  PreSTIM/1 -> Mux2/6
  Lmtu0/1 -> Mux2/7
  NMM_w/1 -> Mux2/8
  NMM_A/1 -> Mux2/9
  TACT/1 -> Mux2/10
  TDACT/1 -> Mux2/11
  KPEE/1 -> Mux2/12
  RANKLE/1 -> Mux2/13
  UMAX/1 -> Mux2/14
  NMM force_offset/1 -> Mux1/6
  est_stride_time/1 -> Mux1/7
  K_NMM/1 -> Mux1/8
  FVMAX/1 -> Mux1/9
  K_STIM/1 -> Mux1/10
  EMG_OFFSET/1 -> Mux1/11
  Vmax/1 -> Mux1/12
  Mux3/1 -> Mux1/13
  ED_P_tauMax/1 -> Mux3/1
  ED_P_tauStep/1 -> Mux3/2
  commdelaycycle/1 -> Mux1/14, commdelay_cycle/1
  isModiAdded/1 -> Mux1/15
  Mux4/1 -> Mux1/16
  Pos_Kd/1 -> Mux4/1
  Pos_Ki/1 -> Mux4/2
  alpha/1 -> Mux4/3
  lambda/1 -> Mux4/4
  isPosPID/1 -> Mux4/5
  lrn_tau_err_threshold/1 -> Mux4/6
  learning_shrink_rate/1 -> Mux4/7
  stimDelayCycle/1 -> Mux4/8
  K_swing_follow/1 -> Mux4/9
  r_motor_shaft/1 -> Mux4/10
  maxPlanter/1 -> Mux4/11
  xadjust_ref/1 -> Mux4/12
  y_adjust_ref/1 -> Mux4/13
  planter_low_limit/1 -> Mux4/14
  curve_k2/1 -> Mux4/15
  ABL Ankle Min/1 -> Mux5/1
  ABL Ankle Res/1 -> Mux5/2
  ABL or TBL/1 -> Mux5/3
  Mux5/1 -> User Inputs - AnkleBasedLearning/1
  Mux6/1 -> Mux1/17
  pos_traj_mode/1 -> Mux6/1
  pos_des_1/1 -> Mux6/2
  pos_des_2/1 -> Mux6/3
  peakTorque/1 -> Mux7/1
  peakTime/1 -> Mux7/2
  riseTime/1 -> Mux7/3
  Mux7/1 -> CusHLCParam/1
  dropTime/1 -> Mux7/4
  Kp_earlyswing/1 -> Mux6/4
  oo_dtau_offset/1 -> Mux6/5

== system youhua_1226/CONTROL/Control and Display/learning data read ==
  indices : Inport
  commdelaycycle : Inport  Port=2
  learningMode : Inport  Port=3
  filtered step data read : Subsystem
  filtredLearndingData : Outport
  wires:
  commdelaycycle/1 -> filtered step data read/2(comm delay cycle)
  indices/1 -> filtered step data read/1(indices)
  filtered step data read/1(oldD) -> filtredLearndingData/1
  learningMode/1 -> filtered step data read/3(learningMode)

== system youhua_1226/CONTROL/Control and Display/learning data write ==
  indices : Inport
  stepdata : Inport  Port=2
  learningMode : Inport  Port=3
  filtered step data write : Subsystem
  wires:
  stepdata/1 -> filtered step data write/2(filteredstepdata)
  indices/1 -> filtered step data write/1(indices)
  learningMode/1 -> filtered step data write/3(learningMode)

== system youhua_1226/CONTROL/Control and Display/ooParmSampleHold ==
  In1 : Inport
  Trigger : TriggerPort  TriggerType=either  VariantControl=(inherit)
  MATLAB Function : MATLAB Function  TreatAsAtomicUnit=on
  Out1 : Outport
  wires:
  MATLAB Function/1(y) -> Out1/1
  In1/1 -> MATLAB Function/1(u)

== system youhua_1226/CONTROL/Control and Display/time derivatives  ==
  state vars : Inport
  MATLAB Function2 : MATLAB Function  TreatAsAtomicUnit=on
  Mux : Mux
  Selector4 : Selector  InputPortWidth=52  IndexOptions=Index vector (dialog)  Indices=[5 6 27]  OutputSizes=1
  get ddot torque : Subsystem
  "get desired torque " : Subsystem
  get desired torque 1 : Subsystem
  get desired torque 2 : Subsystem
  state variable delay : UnitDelay  SampleTime=-1
  dots : Outport
  wires:
  Selector4/1 -> MATLAB Function2/1(u)
  MATLAB Function2/1(desired_torque) -> "get desired torque "/1(data)
  MATLAB Function2/3(desired_motor_pos) -> get desired torque 1/1(data)
  "get desired torque "/1(dotdata) -> get ddot torque/1(data), Mux/1
  state vars/1 -> Selector4/1
  get ddot torque/1(dotdata) -> Mux/2
  get desired torque 1/1(dotdata) -> Mux/3
  Mux/1 -> state variable delay/1
  state variable delay/1 -> dots/1
  MATLAB Function2/2(measured_torque) -> get desired torque 2/1(data)
  get desired torque 2/1(dotdata) -> Mux/4

== system youhua_1226/DSpace Sensor Raw Readings/Analog Channels/Preprocessing ==
  raw_signals : Inport
  Abs : Abs
  high_pass : dsparch4/Analog Filter Design  method=Butterworth  filttype=Highpass  N=2  Wlo=20*2*pi  Whi=80  Rp=2  Rs=40
  low_pass : dsparch4/Analog Filter Design  method=Butterworth  filttype=Lowpass  N=2  Wlo=10*2*pi  Whi=80  Rp=2  Rs=40
  e(t) : Outport
  wires:
  Abs/1 -> low_pass/1
  high_pass/1 -> Abs/1
  raw_signals/1 -> high_pass/1
  low_pass/1 -> e(t)/1

== system youhua_1226/DSpace Sensor Raw Readings/Analog Channels/Preprocessing1 ==
  raw_signals : Inport
  Abs : Abs
  high_pass : dsparch4/Analog Filter Design  method=Butterworth  filttype=Highpass  N=2  Wlo=20*2*pi  Whi=80  Rp=2  Rs=40
  low_pass : dsparch4/Analog Filter Design  method=Butterworth  filttype=Lowpass  N=2  Wlo=10*2*pi  Whi=80  Rp=2  Rs=40
  e(t) : Outport
  wires:
  Abs/1 -> low_pass/1
  high_pass/1 -> Abs/1
  raw_signals/1 -> high_pass/1
  low_pass/1 -> e(t)/1

== system youhua_1226/DSpace Sensor Raw Readings/Analog Channels/Preprocessing2 ==
  raw_signals : Inport
  Abs : Abs
  high_pass : dsparch4/Analog Filter Design  method=Butterworth  filttype=Highpass  N=2  Wlo=20*2*pi  Whi=80  Rp=2  Rs=40
  low_pass : dsparch4/Analog Filter Design  method=Butterworth  filttype=Lowpass  N=2  Wlo=10*2*pi  Whi=80  Rp=2  Rs=40
  e(t) : Outport
  wires:
  Abs/1 -> low_pass/1
  high_pass/1 -> Abs/1
  raw_signals/1 -> high_pass/1
  low_pass/1 -> e(t)/1

== system youhua_1226/RTI Data/RTI Data Store/RTI Data Store ==
  RTI Data Store : Subsystem  mask(RTI_DATA_STORE){}
      mask help:
      | RTI Data Store Block. This block is used by RTI to store internal model dependent data. Deleting this block will result in data loss.
      |
      | NEVER DELETE, COPY, OR MODIFY THIS BLOCK!
      mask Help:
      | RTI Data Store Block. This block is used by RTI to store internal model dependent data. Deleting this block will result in data loss.
      | 
      | NEVER DELETE, COPY, OR MODIFY THIS BLOCK!
      mask Display: text(0.5, 0.5, ' ', 'HorizontalAlignment', 'center');
